simulink model "my_pv_system"  (Simulink 8.4)
settings: Solver=ode4  StartTime=0.0  StopTime=inf  FixedStep=1e-6  RelTol=1e-3
libraries: powerlib x31, powerlib_meascontrol x9, opal_lib x5, rtlab x5, simulink x4
Description:
  | Model of a simple control system for use iin training.
settings Model: Creator=Paul Baracos  LastModifiedBy=jiang  BufferReuse=off
settings DataIOCC: SaveOutput=off  SaveTime=off  SignalLoggingName=sigsOut
settings OptimizationCC: BlockReduction=off  BooleanDataType=off  OptimizeBlockIOStorage=off  BufferReuse=off  GlobalBufferReuse=off  ExpressionFolding=off  ExpressionDepthLimit=128  LocalBlockOutputs=off  InitFltsAndDblsToZero=on
settings DebuggingCC: SaveWithParameterizedLinksMsg=none  SignalResolutionControl=TryResolveAllWithWarning  SolverPrmCheckMsg=none  MultiTaskDSMMsg=warning  MultiTaskCondExecSysMsg=none  StateNameClashWarn=none
settings HardwareCC: TargetHWDeviceType=32-bit Generic  TargetUnknown=on  ProdEqTarget=off
settings RTWCC: IncludeERTFirstTime=on
settings GRTTargetCC: TargetFcnLib=ansi_tfl_tmw.mat

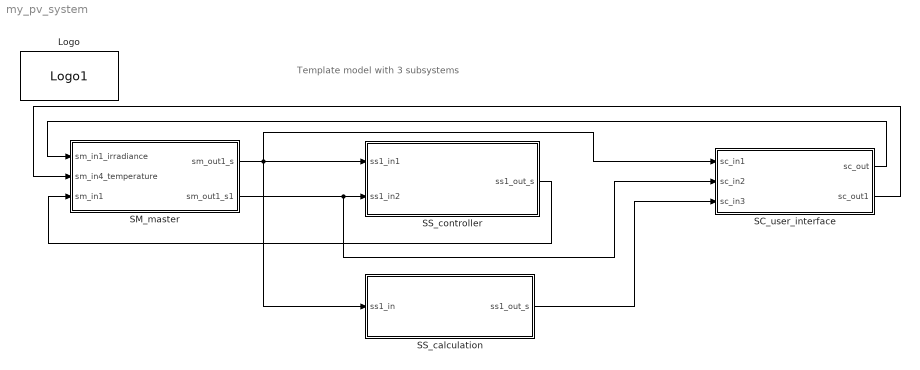
== system my_pv_system ==
  note: Template model with 3 subsystems
  Logo : opal_lib/Logo1  vide=[]
  SC_user_interface : Subsystem
  SM_master : Subsystem
  SS_calculation : Subsystem
  SS_controller : Subsystem
  wires:
  SC_user_interface/1(sc_out) -> SM_master/1(sm_in1_irradiance)
  SM_master/1(sm_out1_s) -> SC_user_interface/1(sc_in1), SS_calculation/1(ss1_in), SS_controller/1(ss1_in1)
  SM_master/2(sm_out1_s1) -> SC_user_interface/2(sc_in2), SS_controller/2(ss1_in2)
  SS_controller/1(ss1_out_s) -> SM_master/3(sm_in1)
  SC_user_interface/2(sc_out1) -> SM_master/2(sm_in4_temperature)
  SS_calculation/1(ss1_out_s) -> SC_user_interface/3(sc_in3)

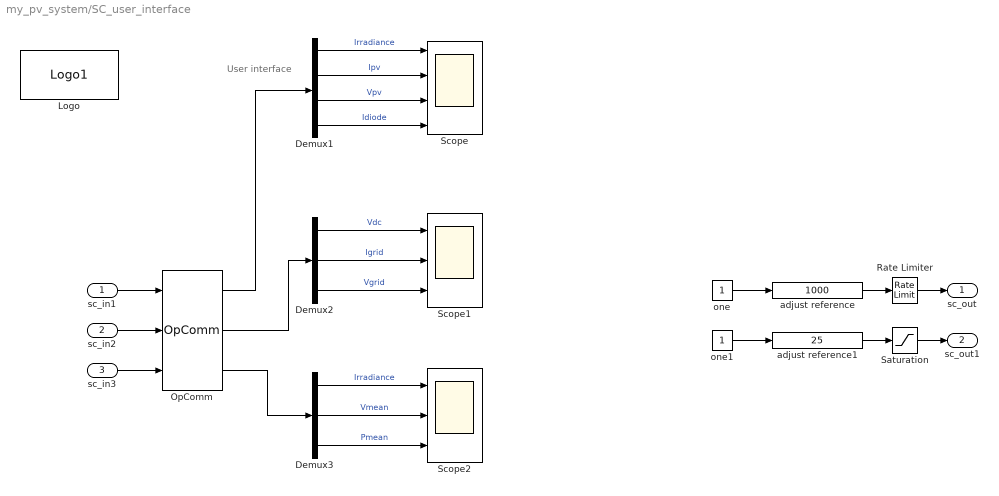
== system my_pv_system/SC_user_interface ==
  note: User interface
  sc_in1 : Inport
  sc_in2 : Inport  Port=2
  sc_in3 : Inport  Port=3
  Demux1 : Demux
  Demux2 : Demux  Outputs=3
  Demux3 : Demux  Outputs=3
  Logo : opal_lib/Logo1  vide=[]
  OpComm : rtlab/OpComm  nbport=3  groupe_acq=1  subsys_rate=0  st=0  Synchronization=on  Interpolation=on  Threshold=1.0  Missed_Data=off  Sim_Time=off  Samples=off  dynSigOut=off  from_console=0  warning_done=off  writeOpCommFile=off  Offset=off
  Rate Limiter : RateLimiter  RisingSlewLimit=8000  FallingSlewLimit=-8000  SampleTimeMode=inherited  InitialCondition=1000
  Saturation : Saturate  UpperLimit=55  LowerLimit=5
  Scope : Scope  NumInputPorts=4
      settings: YMin=0~-5~-5~-5  YMax=100~5~5~5
  Scope1 : Scope  NumInputPorts=3
      settings: YMin=0~-5~-5  YMax=100~5~5
  Scope2 : Scope  NumInputPorts=3
      settings: YMin=0~-5~-5  YMax=100~5~5  SaveName=ScopeData2
  adjust reference : simulink/Math Operations/Slider Gain  low=0  gain=1000  high=1000
  adjust reference1 : simulink/Math Operations/Slider Gain  low=0  gain=25  high=60
  one : Constant
  one1 : Constant
  sc_out : Outport
  sc_out1 : Outport  Port=2
  wires:
  sc_in1/1 -> OpComm/1
  one/1 -> adjust reference/1
  sc_in2/1 -> OpComm/2
  one1/1 -> adjust reference1/1
  sc_in3/1 -> OpComm/3
  Rate Limiter/1 -> sc_out/1
  Saturation/1 -> sc_out1/1
  adjust reference/1 -> Rate Limiter/1
  adjust reference1/1 -> Saturation/1
  OpComm/2 -> Demux2/1
  OpComm/1 -> Demux1/1
  Demux1/2 -> Scope/2  "Ipv"
  Demux1/3 -> Scope/3  "Vpv"
  Demux1/4 -> Scope/4  "Idiode"
  Demux1/1 -> Scope/1  "Irradiance"
  Demux2/2 -> Scope1/2  "Igrid"
  Demux2/3 -> Scope1/3  "Vgrid"
  Demux2/1 -> Scope1/1  "Vdc"
  Demux3/1 -> Scope2/1  "Irradiance"
  Demux3/3 -> Scope2/3  "Pmean"
  Demux3/2 -> Scope2/2  "Vmean"
  OpComm/3 -> Demux3/1

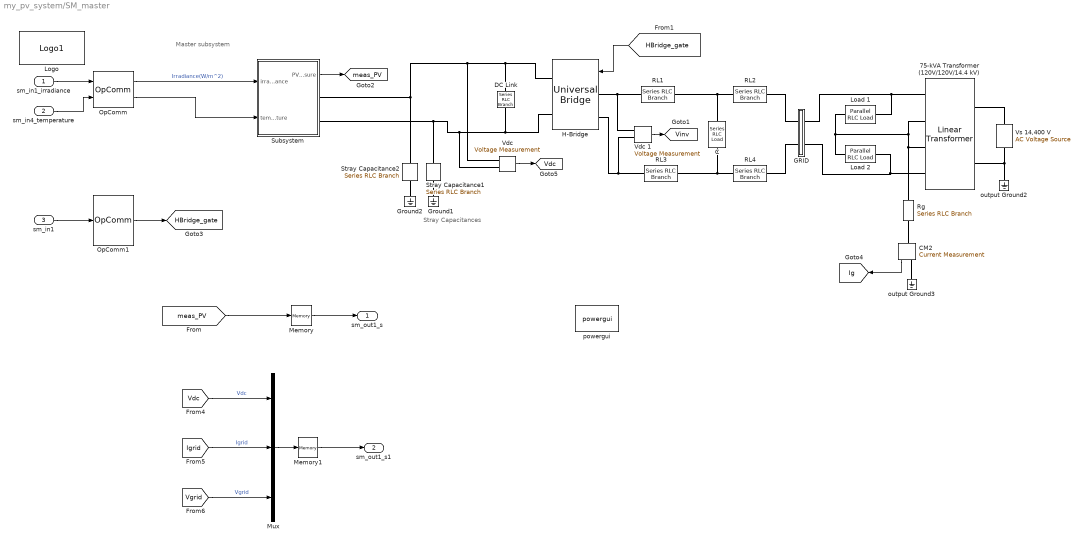
== system my_pv_system/SM_master ==
  note: Master subsystem
  note: Stray
      | Capacitances
  sm_in1_irradiance : Inport
  sm_in4_temperature : Inport  Port=2
  sm_in1 : Inport  Port=3
  75-kVA Transformer (120V/120V/14.4 kV) : powerlib/Elements/Linear Transformer  UNITS=pu  NominalPower=[75e3,60]  winding1=[14.4e3 0.01,0.03]  winding2=[120,0.02,0]  ThreeWindings=on  winding3=[120,0.02,0]  RmLm=[50,50]  Measurements=None  DataType=off
  C : powerlib/Elements/Series RLC Load  LConnTagsString=a  RConnTagsString=__new0  NominalVoltage=240  NominalFrequency=60  ActivePower=10.5  InductivePower=0  CapacitivePower=525  Setx0=off  InitialVoltage=0  SetiL0=off  InitialCurrent=0  Measurements=None
  CM2 : powerlib/Measurements/Current Measurement  PhasorSimulation=off  OutputType=Complex  PSBequivalent=0
  DC Link : powerlib/Elements/Series RLC Branch  LConnTagsString=__new0  RConnTagsString=__new0  BranchType=C  Resistance=1.0  Inductance=1.0  SetiL0=off  InitialCurrent=0  Capacitance=3000e-6  Setx0=on  InitialVoltage=425  Measurements=None
  GRID : Subsystem
  Ground1 : powerlib/Elements/Ground  LConnTagsString=a
  Ground2 : powerlib/Elements/Ground  LConnTagsString=a
  "H-Bridge " : powerlib/Power Electronics/Universal Bridge  Arms=2  SnubberResistance=1e6  SnubberCapacitance=inf  Device=IGBT / Diodes  Ron=1e-3  Lon=0  ForwardVoltages=[ 0 0 ]  ForwardVoltage=0  GTOparameters=[ 10e-6 , 20e-6 ]  IGBTparameters=[ 1e-6 , 2e-6 ]*0  Measurements=None  Measurements_2=None  converterType=Rectifier
  Load 1 : powerlib/Elements/Parallel RLC Load  LConnTagsString=a  RConnTagsString=__new0  NominalVoltage=120  NominalFrequency=50  ActivePower=5e3  InductivePower=2e3  CapacitivePower=0  Setx0=off  InitialVoltage=0  SetiL0=off  InitialCurrent=0  Measurements=None
      settings: AttributesFormatString=\n
  Load 2 : powerlib/Elements/Parallel RLC Load  LConnTagsString=a  RConnTagsString=__new0  NominalVoltage=120  NominalFrequency=50  ActivePower=5e3  InductivePower=2e3  CapacitivePower=0  Setx0=off  InitialVoltage=0  SetiL0=off  InitialCurrent=0  Measurements=None
      settings: AttributesFormatString=\n
  Logo : opal_lib/Logo1  vide=[]
  Memory : Memory  InheritSampleTime=on
  Memory1 : Memory  InheritSampleTime=on
  Mux : Mux  Inputs=3
  OpComm : rtlab/OpComm  nbport=2  groupe_acq=1  subsys_rate=0  st=0  Synchronization=on  Interpolation=on  Threshold=1.0  Missed_Data=off  Sim_Time=off  Samples=off  dynSigOut=off  from_console=1  warning_done=off  writeOpCommFile=off  Offset=off
  OpComm1 : rtlab/OpComm  nbport=1  groupe_acq=1  subsys_rate=0  st=0  Synchronization=on  Interpolation=on  Threshold=1.0  Missed_Data=off  Sim_Time=off  Samples=off  dynSigOut=off  from_console=0  warning_done=off  writeOpCommFile=off  Offset=off
  RL{1..4} (4 alike) : powerlib/Elements/Series RLC Branch  LConnTagsString=__new0  RConnTagsString=__new0  BranchType=RL  Resistance=8.23e-3  Inductance=2.183e-3  SetiL0=off  InitialCurrent=0  Capacitance=1e-6  Setx0=off  InitialVoltage=0  Measurements=None
  Rg : powerlib/Elements/Series RLC Branch  LConnTagsString=__new0  RConnTagsString=__new0  BranchType=R  Resistance=0.2  Inductance=1  SetiL0=off  InitialCurrent=0  Capacitance=50e-9  Setx0=off  InitialVoltage=0  Measurements=None
  Stray Capacitance1 : powerlib/Elements/Series RLC Branch  LConnTagsString=__new0  RConnTagsString=__new0  BranchType=C  Resistance=1e-3  Inductance=1  SetiL0=off  InitialCurrent=0  Capacitance=4e-9  Setx0=off  InitialVoltage=0  Measurements=None
  Stray Capacitance2 : powerlib/Elements/Series RLC Branch  LConnTagsString=__new0  RConnTagsString=__new0  BranchType=C  Resistance=1e-3  Inductance=1  SetiL0=off  InitialCurrent=0  Capacitance=4e-9  Setx0=off  InitialVoltage=0  Measurements=None
  Subsystem : Subsystem
  "Vdc " : powerlib/Measurements/Voltage Measurement  Tag=PoWeRsYsTeMmEaSuReMeNt  PhasorSimulation=off  OutputType=Magnitude  PSBequivalent=0
  Vdc 1 : powerlib/Measurements/Voltage Measurement  Tag=PoWeRsYsTeMmEaSuReMeNt  PhasorSimulation=off  OutputType=Magnitude  PSBequivalent=0
  Vs 14,400 V : powerlib/Electrical Sources/AC Voltage Source  Description=source block  Amplitude=14400*sqrt(2)  Phase=0  Frequency=50  SampleTime=0  Measurements=None
      settings: AttributesFormatString=\n
  output Ground2 : powerlib/Elements/Ground  LConnTagsString=a
  output Ground3 : powerlib/Elements/Ground  LConnTagsString=a
  powergui : powerlib/powergui  Priority=1  SimulationMode=Discrete  SolverType=Tustin/Backward Euler (TBE)  SampleTime=1e-6  frequency=60  SPID=off  DisableSnubberDevices=off  DisableRonSwitches=off  DisableVfSwitches=off  SwTol=0  DisplayEquations=off  Interpol=off  methode=off  Ts=100  frequencyindice=50  Pbase=100e6  ErrMax=1e-4  Iterations=50  UnitsV=kV  UnitsW=MW  FunctionMessages=off  echomessages=off  HookPort=off  EnableUseOfTLC=off  x0status=blocks  RestoreLinks=warning  ResistiveCurrentMeasurement=off  Frange=[0:2:500]  Ylog=off  Xlog=on  ShowGrid=off  save=off  variable=ZData  structure=0  ZoomFFT=off  StartTime=0.0  cycles=1  DisplayStyle=1  fundamental=60  FreqAxis=off  MaxFrequency=1000  frequencyindicesteady=1  RmsSteady=1  display=off
  sm_out1_s : Outport
  sm_out1_s1 : Outport  Port=2
  tag scope: HBridge_gate=global, Ig=global, Vdc=global, Vinv=global, meas_PV=global
  wires:
  sm_in1_irradiance/1 -> OpComm/1
  Memory/1 -> sm_out1_s/1
  sm_in4_temperature/1 -> OpComm/2
  sm_in1/1 -> OpComm1/1
  Vdc 1/1 -> [Vinv]
  "Vdc "/1 -> [Vdc]
  Subsystem/1(PVmeasure) -> [meas_PV]
  OpComm/1 -> Subsystem/1(irradiance)  "Irradiance(W/m^2)"
  OpComm/2 -> Subsystem/2(temperature)
  [meas_PV] -> Memory/1
  OpComm1/1 -> [HBridge_gate]
  [HBridge_gate] -> "H-Bridge "/1
  CM2/1 -> [Ig]
  Memory1/1 -> sm_out1_s1/1
  [Vdc] -> Mux/1  "Vdc"
  [Igrid] -> Mux/2  "Igrid"
  [Vgrid] -> Mux/3  "Vgrid"
  Mux/1 -> Memory1/1
  connections:
  Subsystem/RConn1 -- Stray Capacitance2/LConn1 -- "Vdc "/LConn1 -- DC Link/LConn1 -- "H-Bridge "/RConn1
  RL1/LConn1 -- "H-Bridge "/LConn1 -- Vdc 1/LConn1
  Vdc 1/LConn2 -- "H-Bridge "/LConn2 -- RL3/LConn1
  C/RConn1 -- RL1/RConn1 -- RL2/LConn1
  RL4/LConn1 -- C/LConn1 -- RL3/RConn1
  DC Link/RConn1 -- "H-Bridge "/RConn2 -- Subsystem/RConn2 -- Stray Capacitance1/LConn1 -- "Vdc "/LConn2
  75-kVA Transformer (120V/120V/14.4 kV)/LConn2 -- output Ground2/LConn1 -- Vs 14,400 V/LConn1
  75-kVA Transformer (120V/120V/14.4 kV)/RConn4 -- Load 2/RConn1 -- GRID/RConn2
  75-kVA Transformer (120V/120V/14.4 kV)/RConn1 -- Load 1/RConn1 -- GRID/RConn1
  Load 2/LConn1 -- Load 1/LConn1 -- 75-kVA Transformer (120V/120V/14.4 kV)/RConn2 -- Rg/LConn1 -- 75-kVA Transformer (120V/120V/14.4 kV)/RConn3
  RL2/RConn1 -- GRID/LConn1
  RL4/RConn1 -- GRID/LConn2
  Ground2/LConn1 -- Stray Capacitance2/RConn1
  Vs 14,400 V/RConn1 -- 75-kVA Transformer (120V/120V/14.4 kV)/LConn1
  Ground1/LConn1 -- Stray Capacitance1/RConn1
  CM2/RConn1 -- output Ground3/LConn1
  CM2/LConn1 -- Rg/RConn1

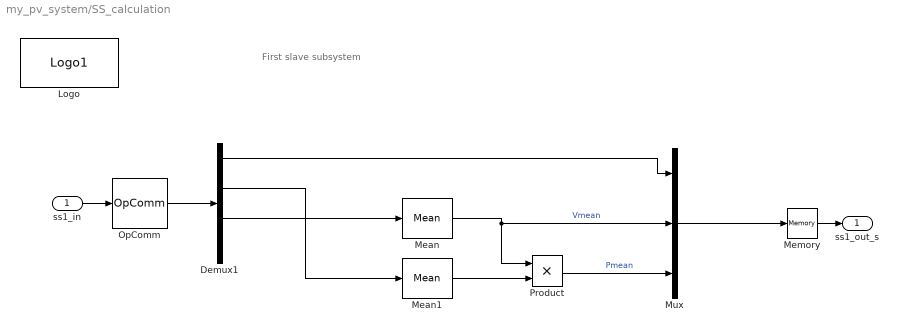
== system my_pv_system/SS_calculation ==
  note: First slave subsystem
  ss1_in : Inport
  Demux1 : Demux
  Logo : opal_lib/Logo1  vide=[]
  Mean : powerlib_meascontrol/Measurements/Mean  Freq=50  Vinit=406  Ts=1e-6
  Mean1 : powerlib_meascontrol/Measurements/Mean  Freq=50  Vinit=8.05  Ts=1e-6
  Memory : Memory  InheritSampleTime=on
  Mux : Mux  Inputs=3
  OpComm : rtlab/OpComm  nbport=1  groupe_acq=1  subsys_rate=0  st=0  Synchronization=on  Interpolation=on  Threshold=1.0  Missed_Data=off  Sim_Time=off  Samples=off  dynSigOut=off  from_console=0  warning_done=off  writeOpCommFile=off  Offset=off
  Product : Product
  ss1_out_s : Outport
  wires:
  Memory/1 -> ss1_out_s/1
  ss1_in/1 -> OpComm/1
  Mean/1 -> Product/1, Mux/2  "Vmean"
  Mean1/1 -> Product/2
  Product/1 -> Mux/3  "Pmean"
  OpComm/1 -> Demux1/1
  Demux1/2 -> Mean1/1
  Demux1/3 -> Mean/1
  Demux1/1 -> Mux/1
  Mux/1 -> Memory/1

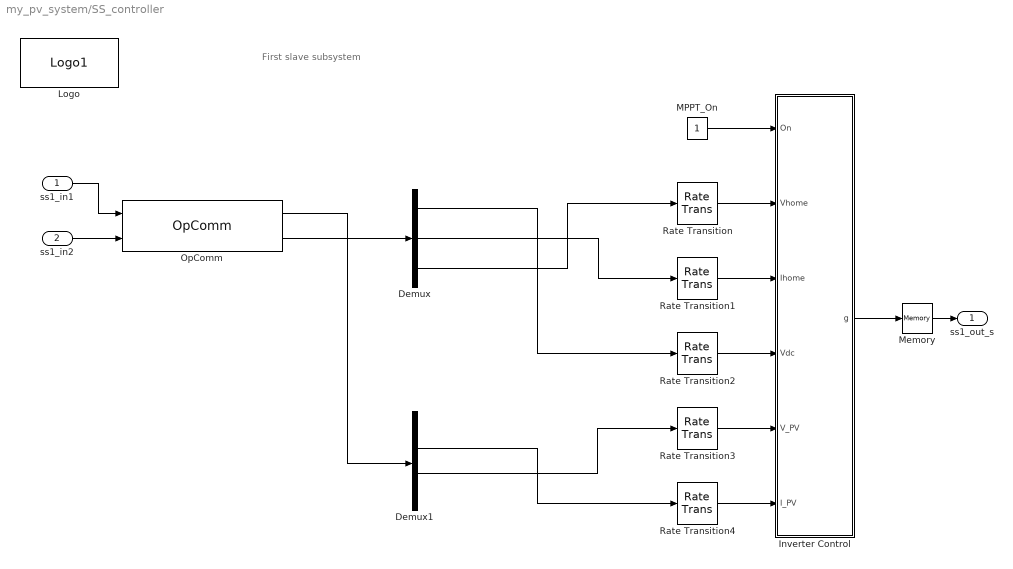
== system my_pv_system/SS_controller ==
  note: First slave subsystem
  ss1_in1 : Inport
  ss1_in2 : Inport  Port=2
  Demux : Demux  Outputs=3
  Demux1 : Demux
  Inverter Control : Subsystem  mask(Inverter Control){Pnom=3500, Fnom=50, Vnom_prim=240, Vnom_dc=400, Increment_MPPT=0.003, Limits_MPPT=[ 450 375 ], Vdc_ref_Init=425, Kp_VDCreg=12, Ki_VDCreg=200, Kp_Ireg=0.15, Ki_Ireg=6.6, RLff=[ 0.002 0.20 ], Fc=4000, PWMmode12=Unipolar, Ts_Control=1e-5, Ts_PWMgenerator=1e-6}
      mask prompts: Pnom "Power (VA)"; Fnom "Frequency (Hz)"; Vnom_prim "Primary voltage (Vrms LL)"; Vnom_dc "DC voltage (V)"; Increment_MPPT "Output increment (V)"; Limits_MPPT "Output limits [ Upper  Lower ]"; Vdc_ref_Init "Output initial value (V)"; Kp_VDCreg "Proportional gain"; Ki_VDCreg "Integral gain"; Kp_Ireg "Proportional gain"; Ki_Ireg "Integral gain"; RLff "Feedforward Values [Rff Lff] (pu)"; Fc "Carrier frequency (Hz)"; PWMmode12 "PWM method"; Ts_Control "Control systems"; Ts_PWMgenerator "PWM generator"
      mask help:
      | The main components of the Inverter Control are:
      | 1. PLL & Measurements
      | 2. Maximum Power Point Tracker System (MPPT) using a Perturb & Observe algorithm
      | 3. DC Voltage Regulator
      | 4. Current Regulator
      | 5. PWM Modulator
      mask init:
      | blockName=gcb;
      | if PWMmode12==1
      |     set_param([blockName,'/','PWM_Generator'],'ModulatorType','Single-phase full-bridge (4 pulses)')
      | else
      |     set_param([blockName,'/','PWM_Generator'],'ModulatorType','Single-phase full-bridge - Bipolar modulation (4 pulses)')
      | end
      mask TypeOptions PWMmode12: Unipolar | Bipolar
  Logo : opal_lib/Logo1  vide=[]
  MPPT_On : Constant
  Memory : Memory  InheritSampleTime=on
  OpComm : rtlab/OpComm  nbport=2  groupe_acq=1  subsys_rate=0  st=0  Synchronization=on  Interpolation=on  Threshold=1.0  Missed_Data=off  Sim_Time=off  Samples=off  dynSigOut=off  from_console=0  warning_done=off  writeOpCommFile=off  Offset=off
  Rate Transition{,1..4} (5 alike) : RateTransition
  ss1_out_s : Outport
  wires:
  Memory/1 -> ss1_out_s/1
  ss1_in1/1 -> OpComm/1
  ss1_in2/1 -> OpComm/2
  MPPT_On/1 -> Inverter Control/1(On)
  Inverter Control/1(g) -> Memory/1
  Rate Transition/1 -> Inverter Control/2(Vhome)
  Rate Transition1/1 -> Inverter Control/3(Ihome)
  Rate Transition2/1 -> Inverter Control/4(Vdc)
  Rate Transition3/1 -> Inverter Control/5(V_PV)
  Rate Transition4/1 -> Inverter Control/6(I_PV)
  OpComm/2 -> Demux/1
  Demux/1 -> Rate Transition2/1
  Demux/2 -> Rate Transition1/1
  Demux/3 -> Rate Transition/1
  OpComm/1 -> Demux1/1
  Demux1/2 -> Rate Transition4/1
  Demux1/3 -> Rate Transition3/1

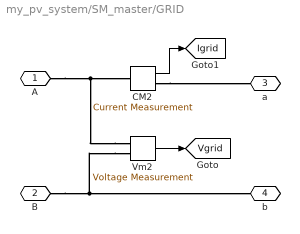
== system my_pv_system/SM_master/GRID ==
  CM2 : powerlib/Measurements/Current Measurement  PhasorSimulation=off  OutputType=Complex  PSBequivalent=0
  Vm2 : powerlib/Measurements/Voltage Measurement  PhasorSimulation=off  OutputType=Complex  PSBequivalent=0
  A : PMIOPort  Port=1  Side=Left
  B : PMIOPort  Port=2  Side=Left
  a : PMIOPort  Port=3  Side=Right
  b : PMIOPort  Port=4  Side=Right
  tag scope: Igrid=global, Vgrid=global
  wires:
  Vm2/1 -> [Vgrid]
  CM2/1 -> [Igrid]
  connections:
  Vm2/LConn2 -- b/RConn1 -- B/RConn1
  Vm2/LConn1 -- A/RConn1 -- CM2/LConn1
  CM2/RConn1 -- a/RConn1

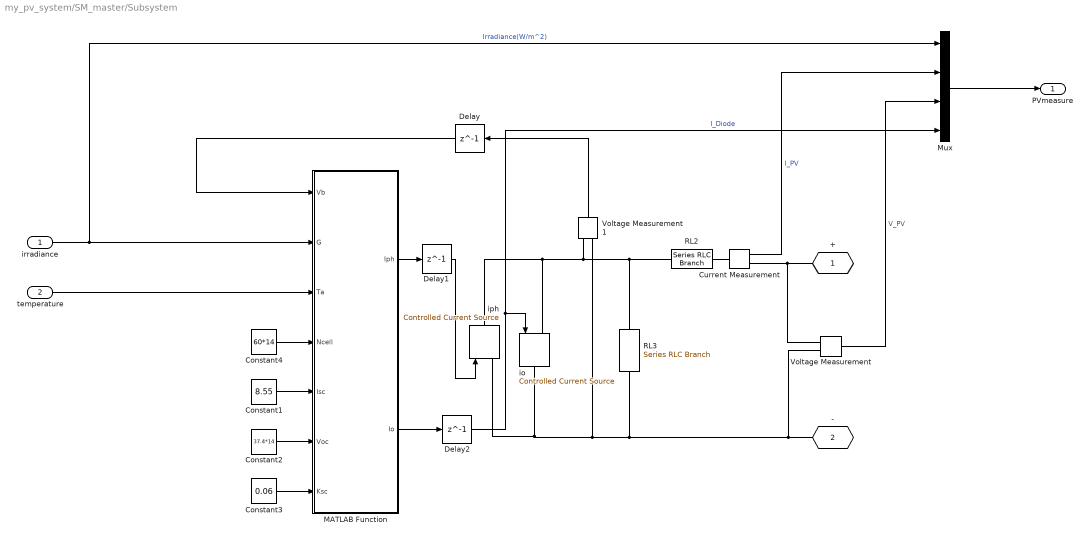
== system my_pv_system/SM_master/Subsystem ==
  irradiance : Inport
  temperature : Inport  Port=2
  Constant1 : Constant  Value=8.55
  Constant2 : Constant  Value=37.4*14
  Constant3 : Constant  Value=0.06
  Constant4 : Constant  Value=60*14
  Current Measurement : powerlib/Measurements/Current Measurement  PhasorSimulation=off  OutputType=Complex  PSBequivalent=0
  Delay : Delay  DelayLength=1  InitialCondition=37.4*14
  Delay1 : Delay  DelayLength=1  InitialCondition=0
  Delay2 : Delay  DelayLength=1  InitialCondition=0
  MATLAB Function : MATLAB Function  TreatAsAtomicUnit=on
  Mux : Mux
  RL2 : powerlib/Elements/Series RLC Branch  LConnTagsString=__new0  RConnTagsString=__new0  BranchType=R  Resistance=0.247*14  Inductance=2.183e-3  SetiL0=off  InitialCurrent=0  Capacitance=1e-6  Setx0=off  InitialVoltage=0  Measurements=None
  RL3 : powerlib/Elements/Series RLC Branch  LConnTagsString=__new0  RConnTagsString=__new0  BranchType=R  Resistance=301.8*14  Inductance=2.183e-3  SetiL0=off  InitialCurrent=0  Capacitance=1e-6  Setx0=off  InitialVoltage=0  Measurements=None
  Voltage Measurement : powerlib/Measurements/Voltage Measurement  PhasorSimulation=off  OutputType=Complex  PSBequivalent=0
  Voltage Measurement1 : powerlib/Measurements/Voltage Measurement  PhasorSimulation=off  OutputType=Complex  PSBequivalent=0
  "io " : powerlib/Electrical Sources/Controlled Current Source  Initialize=on  Source_Type=DC  Amplitude=8.05  Phase=0  Frequency=0  Measurements=None
  "iph " : powerlib/Electrical Sources/Controlled Current Source  Initialize=on  Source_Type=DC  Amplitude=8.05  Phase=0  Frequency=0  Measurements=None
  + : PMIOPort  Port=1  Side=Right
  - : PMIOPort  Port=2  Side=Right
  PVmeasure : Outport
  wires:
  irradiance/1 -> Mux/1, MATLAB Function/2(G)  "Irradiance(W/m^2)"
  temperature/1 -> MATLAB Function/3(Ta)
  Constant4/1 -> MATLAB Function/4(Ncell)
  Constant1/1 -> MATLAB Function/5(Isc)
  Constant2/1 -> MATLAB Function/6(Voc)
  Constant3/1 -> MATLAB Function/7(Ksc)
  Voltage Measurement/1 -> Mux/3  "V_PV"
  Current Measurement/1 -> Mux/2  "I_PV"
  Voltage Measurement1/1 -> Delay/1
  Delay/1 -> MATLAB Function/1(Vb)
  Mux/1 -> PVmeasure/1
  MATLAB Function/1(Iph) -> Delay1/1
  Delay1/1 -> "iph "/1
  MATLAB Function/2(Io) -> Delay2/1
  Delay2/1 -> Mux/4, "io "/1  "I_Diode"
  connections:
  "iph "/RConn1 -- "io "/LConn1 -- RL3/RConn1 -- RL2/LConn1 -- Voltage Measurement1/LConn1
  "io "/RConn1 -- "iph "/LConn1 -- Voltage Measurement/LConn2 -- -/RConn1 -- RL3/LConn1 -- Voltage Measurement1/LConn2
  Current Measurement/LConn1 -- RL2/RConn1
  Current Measurement/RConn1 -- Voltage Measurement/LConn1 -- +/RConn1

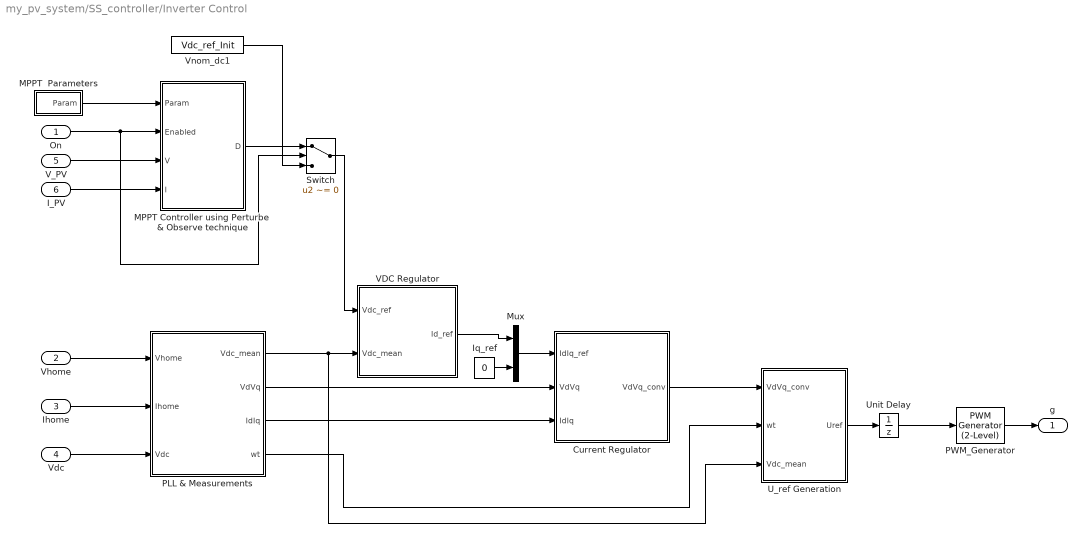
== system my_pv_system/SS_controller/Inverter Control ==
  On : Inport  PortDimensions=1
  Vhome : Inport  Port=2  PortDimensions=1
  Ihome : Inport  Port=3  PortDimensions=1
  Vdc : Inport  Port=4  PortDimensions=1
  V_PV : Inport  Port=5  PortDimensions=1
  I_PV : Inport  Port=6  PortDimensions=1
  Current Regulator : Subsystem
  Iq_ref : Constant  Value=0
  MPPT  Parameters : Subsystem
  "MPPT Controller using Perturbe  & Observe technique  " : MATLAB Function  TreatAsAtomicUnit=on
  Mux : Mux  Inputs=2
  PLL & Measurements : Subsystem
  PWM_Generator : powerlib_meascontrol/Pulse & Signal Generators/PWM Generator (2-Level)  ModulatorType=Single-phase full-bridge (4 pulses)  ModulatorMode=Unsynchronized  Fc=Fc  Pc=90  nF=27  MinMax="[ -1  1 ]"  SamplingTechnique=Natural  ModulatingSignals=off  m=0.8  Freq=60  Phase=0  Ts=Ts_PWMgenerator  ShowCarrierOutport=off
      settings: AttributesFormatString=%<ModulatorType>
  Switch : Switch  Criteria=u2 ~= 0
  "U_ref Generation " : Subsystem
  Unit Delay : UnitDelay  InitialCondition=0.1684  SampleTime=Ts_Control
  VDC Regulator : Subsystem
  Vnom_dc1 : Constant  Value=Vdc_ref_Init
  g : Outport
  wires:
  Iq_ref/1 -> Mux/2
  Vhome/1 -> PLL & Measurements/1(Vhome)
  Ihome/1 -> PLL & Measurements/2(Ihome)
  V_PV/1 -> "MPPT Controller using Perturbe  & Observe technique  "/3(V)
  I_PV/1 -> "MPPT Controller using Perturbe  & Observe technique  "/4(I)
  MPPT  Parameters/1(Param) -> "MPPT Controller using Perturbe  & Observe technique  "/1(Param)
  On/1 -> "MPPT Controller using Perturbe  & Observe technique  "/2(Enabled), Switch/2
  Unit Delay/1 -> PWM_Generator/1
  "MPPT Controller using Perturbe  & Observe technique  "/1(D) -> Switch/1
  Vdc/1 -> PLL & Measurements/3(Vdc)
  Vnom_dc1/1 -> Switch/3
  PLL & Measurements/2(VdVq) -> Current Regulator/2(VdVq)
  PLL & Measurements/3(IdIq) -> Current Regulator/3(IdIq)
  Mux/1 -> Current Regulator/1(IdIq_ref)
  VDC Regulator/1(Id_ref) -> Mux/1
  PLL & Measurements/1(Vdc_mean) -> "U_ref Generation "/3(Vdc_mean), VDC Regulator/2(Vdc_mean)
  Current Regulator/1(VdVq_conv) -> "U_ref Generation "/1(VdVq_conv)
  PLL & Measurements/4(wt) -> "U_ref Generation "/2(wt)
  "U_ref Generation "/1(Uref) -> Unit Delay/1
  PWM_Generator/1 -> g/1
  Switch/1 -> VDC Regulator/1(Vdc_ref)

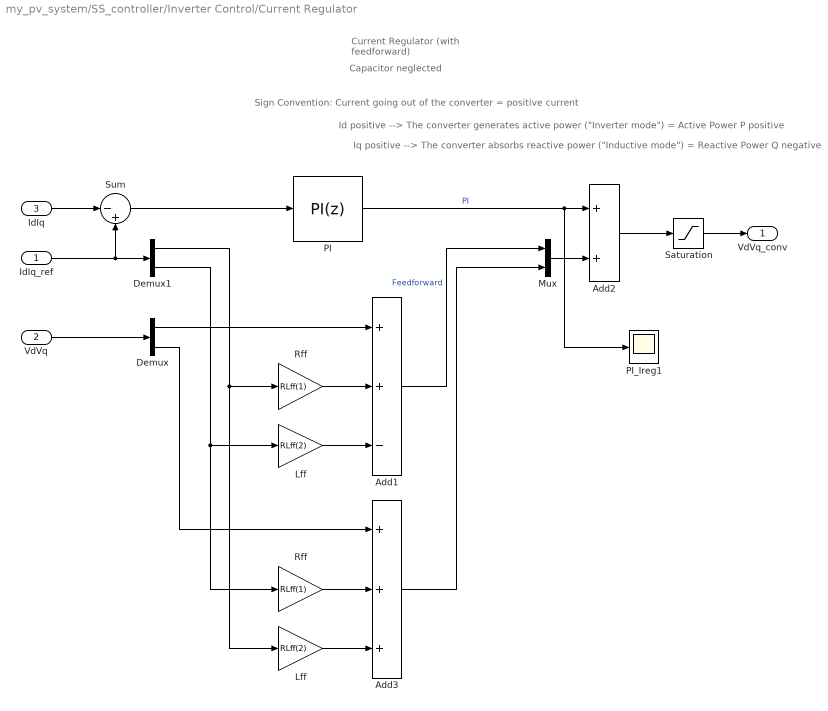
== system my_pv_system/SS_controller/Inverter Control/Current Regulator ==
  note: Id positive --> The converter generates active power ("Inverter mode") = Active Power P positive
  note: Iq positive --> The converter absorbs reactive power ("Inductive mode") = Reactive Power Q negative
  note: Sign Convention: Current going out of the converter = positive current
  note: Current Regulator
      | (with feedforward)
  note: Capacitor neglected
  IdIq_ref : Inport  PortDimensions=2
  VdVq : Inport  Port=2  PortDimensions=2
  IdIq : Inport  Port=3  PortDimensions=2
  Add1 : Sum  Inputs=++-
  Add2 : Sum
  Add3 : Sum  Inputs=+++
  Demux : Demux  Outputs=2
  Demux1 : Demux  Outputs=2
  Lff : Gain  Gain=RLff(2)  SaturateOnIntegerOverflow=on  OutDataTypeStr=Inherit: Same as input  ParamDataTypeStr=Inherit: Same as input
  "Lff  " : Gain  Gain=RLff(2)  SaturateOnIntegerOverflow=on  OutDataTypeStr=Inherit: Same as input  ParamDataTypeStr=Inherit: Same as input
  Mux : Mux  Inputs=2
  PI : simulink/Continuous/PID Controller  Controller=PI  TimeDomain=Discrete-time  SampleTime=Ts_Control  IntegratorMethod=Forward Euler  FilterMethod=Forward Euler  Form=Parallel  P=Kp_Ireg  I=Ki_Ireg  D=0  N=100  InitialConditionSource=internal  InitialConditionForIntegrator=0  InitialConditionForFilter=0  ExternalReset=none  LimitOutput=on  UpperSaturationLimit=1.5  LowerSaturationLimit=-1.5  LinearizeAsGain=off  AntiWindupMode=none  Kb=1  TrackingMode=off  Kt=1  PParamMin=[]  PParamMax=[]  IParamMin=[]  IParamMax=[]  DParamMin=[]  DParamMax=[]  NParamMin=[]  NParamMax=[]  KbParamMin=[]  KbParamMax=[]  KtParamMin=[]  KtParamMax=[]  POutMin=[]  POutMax=[]  IOutMin=[]  IOutMax=[]  DOutMin=[]  DOutMax=[]  NOutMin=[]  NOutMax=[]  KbOutMin=[]  KbOutMax=[]  KtOutMin=[]  KtOutMax=[]  IntegratorOutMin=[]  IntegratorOutMax=[]  FilterOutMin=[]  FilterOutMax=[]  SumOutMin=[]  SumOutMax=[]  SumI1OutMin=[]  SumI1OutMax=[]  SumI2OutMin=[]  SumI2OutMax=[]  SumI3OutMin=[]  SumI3OutMax=[]  SumDOutMin=[]  SumDOutMax=[]  SaturationOutMin=[]  SaturationOutMax=[]  IntegratorContinuousStateAttributes=''  IntegratorStateMustResolveToSignalObject=off  IntegratorRTWStateStorageClass=Auto  FilterContinuousStateAttributes=''  FilterStateMustResolveToSignalObject=off  FilterRTWStateStorageClass=Auto  DifferentiatorICPrevScaledInput=0  DifferentiatorOutMin=[]  DifferentiatorOutMax=[]  UseFilter=on
  PI_Ireg1 : Scope
      settings: YMin=-0.25  YMax=0.45
  Rff : Gain  Gain=RLff(1)  SaturateOnIntegerOverflow=on  OutDataTypeStr=Inherit: Same as input  ParamDataTypeStr=Inherit: Same as input
  "Rff " : Gain  Gain=RLff(1)  SaturateOnIntegerOverflow=on  OutDataTypeStr=Inherit: Same as input  ParamDataTypeStr=Inherit: Same as input
  Saturation : Saturate  UpperLimit=1.5  LowerLimit=-1.5
  Sum : Sum  Inputs=|-+
  VdVq_conv : Outport
  wires:
  Add3/1 -> Mux/2
  Demux/2 -> Add3/1
  Add1/1 -> Mux/1  "Feedforward"
  Lff/1 -> Add3/3
  Rff/1 -> Add3/2
  Demux1/2 -> Rff/1, "Lff  "/1
  "Lff  "/1 -> Add1/3
  Demux1/1 -> Lff/1, "Rff "/1
  "Rff "/1 -> Add1/2
  Demux/1 -> Add1/1
  VdVq/1 -> Demux/1
  Saturation/1 -> VdVq_conv/1
  Add2/1 -> Saturation/1
  IdIq/1 -> Sum/1
  IdIq_ref/1 -> Demux1/1, Sum/2
  Sum/1 -> PI/1
  PI/1 -> Add2/1, PI_Ireg1/1  "PI"
  Mux/1 -> Add2/2

== system my_pv_system/SS_controller/Inverter Control/MPPT  Parameters ==
  note: Upper limit for Vdc_ref (Dmax)
  note: Increment value used to increase/decrease Vdc_ref (DeltaD)
  note: Initial value for Vdc_ref output (Dinit)
  note: Lower limit for Vdc_ref (Dmax)
  note: Parameters for Perturb and Observe Algorithm:
  Iph_ : Constant  Value=Vdc_ref_Init
  Iph_1 : Constant  Value=Limits_MPPT(1)
  Iph_2 : Constant  Value=Limits_MPPT(2)
  Iph_3 : Constant  Value=Increment_MPPT
  Mux : Mux
  Param : Outport
  wires:
  Iph_/1 -> Mux/1
  Iph_1/1 -> Mux/2
  Iph_2/1 -> Mux/3
  Iph_3/1 -> Mux/4
  Mux/1 -> Param/1

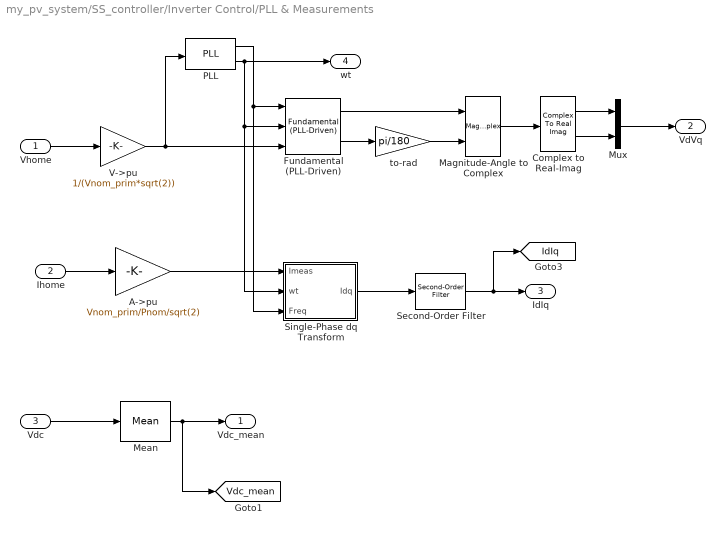
== system my_pv_system/SS_controller/Inverter Control/PLL & Measurements ==
  Vhome : Inport
  Ihome : Inport  Port=2
  Vdc : Inport  Port=3
  A->pu : Gain  Gain=Vnom_prim/Pnom/sqrt(2)  SaturateOnIntegerOverflow=on  OutDataTypeStr=Inherit: Same as input  ParamDataTypeStr=Inherit: Same as input
  Complex to Real-Imag : ComplexToRealImag
  Fundamental (PLL-Driven) : powerlib_meascontrol/Measurements/Fundamental (PLL-Driven)  Finit=Fnom  Fmin=45  InInit=[1, 0]  Ts=Ts_Control
  Magnitude-Angle to Complex : MagnitudeAngleToComplex
  Mean : powerlib_meascontrol/Measurements/Mean  Freq=Fnom  Vinit=Vdc_ref_Init  Ts=Ts_Control
  Mux : Mux  Inputs=2
  PLL : powerlib_meascontrol/PLL/PLL  Fmin=40  Par_Init=[0, Fnom]  ParK=[180, 3200, 1]  TcD=1e-4  MaxRateChangeFreq=12  FilterCutOffFreq=25  Ts=Ts_Control  AGC=on
  Second-Order Filter : powerlib_meascontrol/Filters/Second-Order Filter  FilterType=Lowpass  Fo=2000  Zeta=1  Ts=Ts_Control  Initialize=on  Vac_Init="[0,  0,  60;0,0,60]"  Vdc_Init=[0.9 0]  PlotResponse=off  FreqRange=[0, 500, 1]
  Single-Phase dq Transform : Subsystem
  V->pu : Gain  Gain=1/(Vnom_prim*sqrt(2))  SaturateOnIntegerOverflow=on  OutDataTypeStr=Inherit: Same as input  ParamDataTypeStr=Inherit: Same as input
  to-rad : Gain  Gain=pi/180
  Vdc_mean : Outport
  VdVq : Outport  Port=2
  IdIq : Outport  Port=3
  wt : Outport  Port=4
  tag scope: IdIq=global, Vdc_mean=global
  wires:
  Mean/1 -> Vdc_mean/1, [Vdc_mean]
  Vdc/1 -> Mean/1
  to-rad/1 -> Magnitude-Angle to Complex/2
  Mux/1 -> VdVq/1
  Complex to Real-Imag/2 -> Mux/2
  Complex to Real-Imag/1 -> Mux/1
  Magnitude-Angle to Complex/1 -> Complex to Real-Imag/1
  Fundamental (PLL-Driven)/2 -> to-rad/1
  Fundamental (PLL-Driven)/1 -> Magnitude-Angle to Complex/1
  A->pu/1 -> Single-Phase dq Transform/1(Imeas)
  PLL/1 -> Single-Phase dq Transform/3(Freq), Fundamental (PLL-Driven)/1
  PLL/2 -> wt/1, Fundamental (PLL-Driven)/2, Single-Phase dq Transform/2(wt)
  Ihome/1 -> A->pu/1
  Vhome/1 -> V->pu/1
  V->pu/1 -> Fundamental (PLL-Driven)/3, PLL/1
  Single-Phase dq Transform/1(Idq) -> Second-Order Filter/1
  Second-Order Filter/1 -> [IdIq], IdIq/1

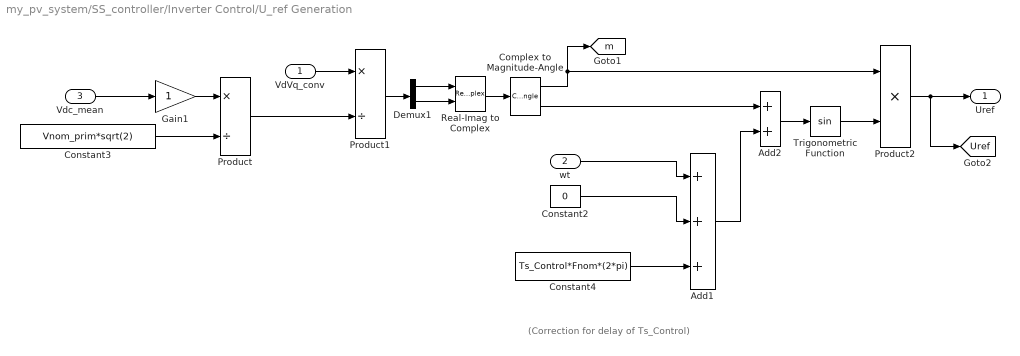
== system my_pv_system/SS_controller/Inverter Control/U_ref Generation  ==
  note: (Correction for delay of Ts_Control)
  VdVq_conv : Inport
  wt : Inport  Port=2
  Vdc_mean : Inport  Port=3
  Add1 : Sum  Inputs=+++
  Add2 : Sum
  Complex to Magnitude-Angle : ComplexToMagnitudeAngle
  Constant2 : Constant  Value=0
  Constant3 : Constant  Value=Vnom_prim*sqrt(2)
  Constant4 : Constant  Value=Ts_Control*Fnom*(2*pi)
  Demux1 : Demux  Outputs=2
  Gain1 : Gain
  Product : Product  Inputs=*/  RndMeth=Zero
  Product1 : Product  Inputs=*/  RndMeth=Zero
  Product2 : Product  Inputs=**  RndMeth=Zero
  Real-Imag to Complex : RealImagToComplex
  Trigonometric Function : Trigonometry
  Uref : Outport
  tag scope: Uref=global, m=global
  wires:
  VdVq_conv/1 -> Product1/1
  Product2/1 -> Uref/1, [Uref]
  Vdc_mean/1 -> Gain1/1
  Constant4/1 -> Add1/3
  wt/1 -> Add1/1
  Trigonometric Function/1 -> Product2/2
  Complex to Magnitude-Angle/1 -> [m], Product2/1
  Add2/1 -> Trigonometric Function/1
  Add1/1 -> Add2/2
  Complex to Magnitude-Angle/2 -> Add2/1
  Product/1 -> Product1/2
  Constant3/1 -> Product/2
  Constant2/1 -> Add1/2
  Demux1/2 -> Real-Imag to Complex/2
  Demux1/1 -> Real-Imag to Complex/1
  Real-Imag to Complex/1 -> Complex to Magnitude-Angle/1
  Gain1/1 -> Product/1
  Product1/1 -> Demux1/1

== system my_pv_system/SS_controller/Inverter Control/VDC Regulator ==
  Vdc_ref : Inport  PortDimensions=1
  Vdc_mean : Inport  Port=2  PortDimensions=1
  PI : simulink/Continuous/PID Controller  Controller=PI  TimeDomain=Discrete-time  SampleTime=Ts_Control  IntegratorMethod=Trapezoidal  FilterMethod=Forward Euler  Form=Parallel  P=Kp_VDCreg  I=Ki_VDCreg  D=0  N=100  InitialConditionSource=internal  InitialConditionForIntegrator=0.9226  InitialConditionForFilter=0  ExternalReset=none  LimitOutput=on  UpperSaturationLimit=1.5  LowerSaturationLimit=-1.5  LinearizeAsGain=off  AntiWindupMode=none  Kb=1  TrackingMode=off  Kt=1  PParamMin=[]  PParamMax=[]  IParamMin=[]  IParamMax=[]  DParamMin=[]  DParamMax=[]  NParamMin=[]  NParamMax=[]  KbParamMin=[]  KbParamMax=[]  KtParamMin=[]  KtParamMax=[]  POutMin=[]  POutMax=[]  IOutMin=[]  IOutMax=[]  DOutMin=[]  DOutMax=[]  NOutMin=[]  NOutMax=[]  KbOutMin=[]  KbOutMax=[]  KtOutMin=[]  KtOutMax=[]  IntegratorOutMin=[]  IntegratorOutMax=[]  FilterOutMin=[]  FilterOutMax=[]  SumOutMin=[]  SumOutMax=[]  SumI1OutMin=[]  SumI1OutMax=[]  SumI2OutMin=[]  SumI2OutMax=[]  SumI3OutMin=[]  SumI3OutMax=[]  SumDOutMin=[]  SumDOutMax=[]  SaturationOutMin=[]  SaturationOutMax=[]  IntegratorContinuousStateAttributes=''  IntegratorStateMustResolveToSignalObject=off  IntegratorRTWStateStorageClass=Auto  FilterContinuousStateAttributes=''  FilterStateMustResolveToSignalObject=off  FilterRTWStateStorageClass=Auto  DifferentiatorICPrevScaledInput=0  DifferentiatorOutMin=[]  DifferentiatorOutMax=[]  UseFilter=on
  Rtot_pu2 : Gain  Gain=1/Vnom_dc  SaturateOnIntegerOverflow=on  OutDataTypeStr=Inherit: Same as input  ParamDataTypeStr=Inherit: Same as input
  Sum : Sum  Inputs=|+-
  Id_ref : Outport  InitialOutput=0
  tag scope: Id_ref=global, Vdc_ref=global
  wires:
  Rtot_pu2/1 -> PI/1
  Vdc_ref/1 -> Sum/2, [Vdc_ref]
  Vdc_mean/1 -> Sum/1
  Sum/1 -> Rtot_pu2/1
  PI/1 -> Id_ref/1, [Id_ref]

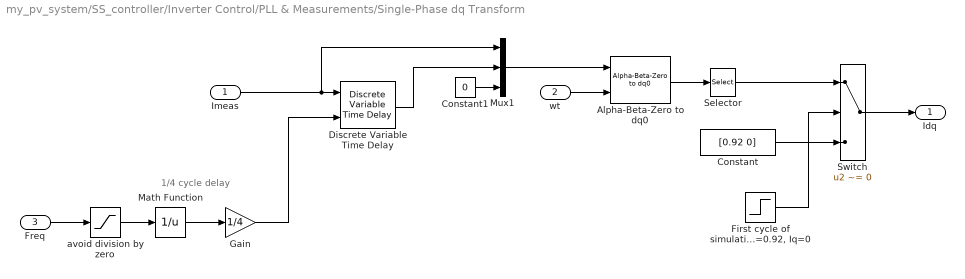
== system my_pv_system/SS_controller/Inverter Control/PLL & Measurements/Single-Phase dq Transform ==
  note: 1/4 cycle delay
  Imeas : Inport
  wt : Inport  Port=2
  Freq : Inport  Port=3
  Alpha-Beta-Zero to dq0 : powerlib_meascontrol/Transformations/Alpha-Beta-Zero to dq0  Alignment=90 degrees behind phase A axis
  Constant : Constant  Value=[0.92 0]
  Constant1 : Constant  Value=0
  Discrete Variable Time Delay : powerlib_meascontrol/Additional Components/Discrete Variable Time Delay  MaxDelay=1  InitialValue=0  Ts=Ts_Control  DFT=on
  "First cycle of simulation Id=0.92, Iq=0" : Step  Time=1/Fnom  SampleTime=Ts_Control
  Gain : Gain  Gain=1/4
  Math Function : Math  Operator=reciprocal  SaturateOnIntegerOverflow=on
  Mux1 : Mux  Inputs=3
  Selector : Selector  InputPortWidth=3  Indices=[1 2]
  Switch : Switch  Criteria=u2 ~= 0
  avoid division by zero : Saturate  UpperLimit=70  LowerLimit=40
  Idq : Outport
  wires:
  Constant1/1 -> Mux1/3
  Discrete Variable Time Delay/1 -> Mux1/2
  Mux1/1 -> Alpha-Beta-Zero to dq0/1
  Imeas/1 -> Discrete Variable Time Delay/1, Mux1/1
  wt/1 -> Alpha-Beta-Zero to dq0/2
  Alpha-Beta-Zero to dq0/1 -> Selector/1
  Freq/1 -> avoid division by zero/1
  avoid division by zero/1 -> Math Function/1
  Math Function/1 -> Gain/1
  Gain/1 -> Discrete Variable Time Delay/2
  Selector/1 -> Switch/1
  Switch/1 -> Idq/1
  Constant/1 -> Switch/3
  "First cycle of simulation Id=0.92, Iq=0"/1 -> Switch/2

== matlab function SM_master/Subsystem/MATLAB Function ==
  data: Vb input double; Iph output double; G input double; Ta input double; Ncell input double; Isc input double; Voc input double; Ksc input double; Io output double
function [Iph, Io] = PVpanel_new(Vb, G, Ta, Ncell, Isc, Voc, Ksc)

    toKelvin = 273;
    Ksc = Ksc / 100;
    G_ref = 1000;
    Ta_ref = 25 + toKelvin;
    Ta = Ta + toKelvin;
    deltaT = Ta - Ta_ref;
    k = 1.381e-23;
    q = 1.6e-19;
    eg = 1.12;                  % bandgap energy(1.12 eV)
    A = 1.3;                    % ideal factor
    a = Ncell * k * A * Ta / q;
    a_ref = Ncell * k * A * Ta_ref / q;
    Iph_ref = Isc;
    Voc_ref = Voc;
    Iph = G / G_ref * Iph_ref * (1 + Ksc * deltaT);
    Io_ref = Iph_ref / (exp(Voc_ref / a_ref) - 1);
    Io = Io_ref * (Ta / Ta_ref)^3 * ...
        exp((q * eg / A / k) * (1/Ta_ref - 1/Ta));
    Io = Io * (exp(Vb / a) - 1);

end

== matlab function SS_controller/Inverter Control/MPPT Controller using Perturbe & Observe technique  ==
  settings: updateMethod=DISCRETE  sampleTime=Ts_Control
  data: Param input double; Enabled input double; V input double; I input double; D output double
function D  = PandO(Param, Enabled, V, I)

% MPPT controller based on the Perturb & Observe algorithm.

% D output = Reference for DC link voltage (Vdc_ref) 
%
% Enabled input = 1 to enable the MPPT controller
% V input = PV array terminal voltage (V)
% I input = PV array current (A)
%
% Param input:
Dinit = Param(1);  %Initial value for Vdc_ref
Dmax = Param(2);   %Maximum value for Vdc_ref
Dmin = Param(3);   %Minimum value for Vdc_ref
deltaD = Param(4); %Increment value used to increase/decrease Vdc_ref
%  

persistent Vold Pold Dold;

dataType = 'double';

if isempty(Vold)
    Vold=0;
    Pold=0;
    Dold=Dinit;
end
P= V*I;
dV= V - Vold;
dP= P - Pold;

if dP ~= 0 & Enabled ~=0
    if dP < 0
        if dV < 0
            D = Dold + deltaD;
        else
            D = Dold - deltaD;
        end
    else
        if dV < 0
            D = Dold - deltaD;
        else
            D = Dold + deltaD;
        end    
    end
else D=Dold;
end

if D >= Dmax | D<= Dmin
    D=Dold;
end

Dold=D;
Vold=V;
Pold=P;
